simulink model "planta_controlada"  (R2013a)
settings: Solver=ode45  StartTime=0.0  StopTime=10.0  RelTol=1e-3
values from neighbouring files (symbols this model uses):
  A = 0.01*ones(4)    [auxiliar.m]    (also in controleAl4Tanks.m = [0.9393   -0.1778    0.0225    0.0571; controleAl4TanksE1.m = [0.9393   -0.1778    0.0225    0.0571; controleAl4TanksE2.m = [0.9393   -0.1778    0.0225    0.0571; controleAlocacao.m = [0 1 0)
  B = 0.01*ones(4,2)    [auxiliar.m]    (also in controleAl4Tanks.m = [0.0283    0.0196; controleAl4TanksE1.m = [0.0283    0.0196; controleAl4TanksE2.m = [0.0283    0.0196; controleAlocacao.m = [0 0)
  C = eye(4)    [auxiliar.m]    (also in controleAl4TanksE1.m = [1 0 0 0]; controleAl4TanksE2.m = [1 0 0 0; controleAlocacao.m = [1 0 0]; controleAlocacao2.m = [1 0 0)
undefined symbols (not defined in the file or in its folder): Ki, Kp
settings Model: Creator=jhona  LastModifiedBy=jhona

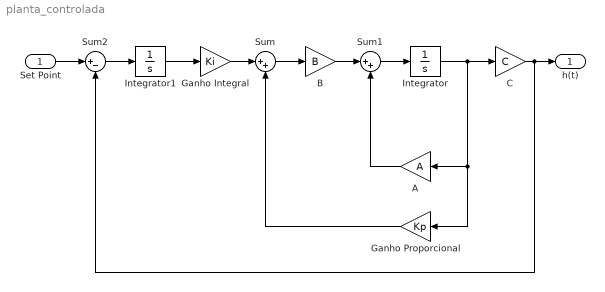
== system planta_controlada ==
  Set Point : Inport
  A : Gain  Gain=A
  B : Gain  Gain=B
  C : Gain  Gain=C
  Ganho Integral : Gain  Gain=Ki
  Ganho Proporcional : Gain  Gain=Kp
  Integrator : Integrator
  Integrator1 : Integrator
  Sum : Sum  Inputs=|++
  Sum1 : Sum  Inputs=|++
  Sum2 : Sum  Inputs=|+-
  h(t) : Outport
  wires:
  Sum/1 -> B/1
  Integrator/1 -> C/1, Ganho Proporcional/1, A/1
  Sum1/1 -> Integrator/1
  B/1 -> Sum1/1
  A/1 -> Sum1/2
  Ganho Proporcional/1 -> Sum/2
  Ganho Integral/1 -> Sum/1
  C/1 -> h(t)/1, Sum2/2
  Sum2/1 -> Integrator1/1
  Integrator1/1 -> Ganho Integral/1
  Set Point/1 -> Sum2/1
